simulink model "rtlsdr_datafm_image_audio"  (R2014b)
settings: Solver=ode45  StartTime=0.0  StopTime=170  RelTol=1e-3
PreLoadFcn:
  | %%%%%%%%%%%%%%%%%%%%%%%%%%%%%%%%%%%%%%%%%%%%%%%%%%%%%%%%%%%%%%%%%%%%%%%%%%%
  | % check to see if Simulink library folder is missing from the MATLAB path %
  | %%%%%%%%%%%%%%%%%%%%%%%%%%%%%%%%%%%%%%%%%%%%%%%%%%%%%%%%%%%%%%%%%%%%%%%%%%%
  | if isempty(strfind(path, 'rtlsdr_book_library'))
  | 
  |     % create error window
  |     fig_error = figure(...
  |         'Name', 'Error: RTL-SDR Book Library',...
  |         'Toolbar','none',...
  |         'MenuBar','none',...
  |         'NumberTitle','off',...
  |         'Resize','off',...
  |         'WindowStyle','modal');
  |     fig_error.Position(3) = 600;
  |     fig_error.Position(4) = 150;
  |     fig_axes = axes(...
  |         'Parent',fig_error,...
  |         'Position',[0,0,1,1],...
  |         'visible','off');
  |     % error message
  |     t_title = text(.05,.8,...
  |         'MISSING DIRECTORIES',...
  |         'FontSize',11.5);
  |     t_body = text(.075,.6,...
  |         [{'Simulink cannot find the  \it{<root>}\rm / \it{rtlsdr\_book\_library}\rm  folder in the \it{MATLAB Path}\rm.'},...
  |         {'Please set the MATLAB path following the instructions given in Exercise 2.4.'}],...
  |         'FontSize',10.5);
  |     % buttons
  |     btn_path = uicontrol(...
  |         'Parent',fig_error,...
  |         'String','Set Path Now',...
  |         'FontSize',10,...
  |         'Callback', 'pathtool; close(fig_error);',...
  |         'Position', [fig_error.Position(3)/2-210, 30, 200, 30]);
  |     btn_abort = uicontrol(...
  |         'Parent',fig_error,...
  |         'String','No thanks',...
  |         'FontSize',10,...
  |         'Callback', 'close(fig_error); abort=1;',...
  |         'Position', [fig_error.Position(3)/2+10, 30, 200, 30]);
  | 
  |     % pause to allow user to interact with error box
  |     uiwait(fig_error);
  | 
  |     % abort simulation
  |     try
  |         if abort==1
  |             set_param(gcs, 'SimulationCommand', 'stop');
  |         end
  |     end
  | 
  |     % if user has set path, allow diagram to be updated
  |     if ~exist('abort','var')
  |         % create error window
  |         fig_update = figure(...
  |             'Name', 'Update Diagram',...
  |             'Toolbar','none',...
  |             'MenuBar','none',...
  |             'NumberTitle','off',...
  |             'Resize','off');
  |         fig_update.Position(3) = 400;
  |         fig_update.Position(4) = 120;
  |         fig_axes = axes(...
  |             'Parent',fig_update,...
  |             'Position',[0,0,1,1],...
  |             'visible','off');
  |         % instruction message
  |         t_body = text(.075,.7,...
  |             'Once you have set the path, update the block diagram',...
  |             'FontSize',10.5);
  |         % button
  |         btn_update = uicontrol(...
  |             'Parent',fig_update,...
  |             'String','Update Block Diagram',...
  |             'FontSize',10,...
  |             'Callback', 'set_param(gcs,''SimulationCommand'',''update''); close(gcf)',...
  |             'Position', [fig_update.Position(3)/2-100, 30, 200, 30]);
  |     end
  | 
  |     % clear error components
  |     clear('fig_error','fig_update','fig_axes','t_title','t_body','btn_path','btn_abort','btn_update','abort');
  | 
  | end
  | %%%%%%%%%%%%%%%%%%%%%%%%%%%%%%%%%%%%%%%%%%%%%%%%%%%%%%%%%%%%%%%%%%%%%%%%%%%
undefined symbols (not defined in the file): dfilt, fdesignblkfcn, frm, gcbh, startfcn_spectrum_analyzer
libraries: simulink x5, dsparch4 x3, rtlsdr_book_library x3, dspmlti4 x2, commutil2 x2, commrfcorlib x1, dspstat3 x1, sdrrlib x1, dspsnks4 x1
CloseFcn:
  | closefcn_model;
Description:
  | Software, Simulation Examples and Design Exercises Licence Agreement
  | 
  | This license agreement refers to the simulation examples, design exercises and files,
  | and associated software MATLAB and Simulink resources that accompany the book:
  | 
  |      Title: Software Defined Radio using MATLAB & Simulink and the RTL-SDR
  |      Published by Strathclyde Academic Media, 2015
  |      Authored by Robert W. Stewart, Kenneth W. Barlee, Dale S.W. Atkinson,
  |      and Louise H. Crockett
  | 
  | and made available as a download from, www.desktopSDR.com or variously acquired
  | by other means such as via USB storage, cloud storage, disk or any other electronic
  | or optical or magnetic storage mechanism. These files and associated software may
  | be used subject to the terms of agreement of the conditions below:
  | 
  |     Copyright © 2015 Robert W. Stewart, Kenneth W. Barlee, Dale S.W. Atkinson,
  |     and Louise H. Crockett
  |     All rights reserved.
  | 
  | Redistribution and use in source and binary forms, with or without modification, are
  | permitted provided that the following conditions are met:
  | 
  |    1.  Redistributions of source code must retain the above copyright notice, this list of
  |         conditions and the following disclaimer.
  | 
  |    2.  Redistributions in binary form must reproduce the above copyright notice, this
  |         list of conditions and the following disclaimer in the documentation and/or other
  |         materials provided with the distribution.
  | 
  |    3.  Neither the name of the copyright holder nor the names of its contributors may
  |         be used to endorse or promote products derived from this software without
  |         specific prior written permission.
  | 
  |    4.  In all cases, the software is, and all modifications and derivatives of the
  |         software shall be, licensed to you solely for use in conjunction with The
  |         MathWorks, Inc. products and service offerings.
  | 
  | THIS SOFTWARE IS PROVIDED BY THE COPYRIGHT HOLDERS AND CONTRIBUTORS
  | "AS IS" AND ANY EXPRESS OR IMPLIED WARRANTIES, INCLUDING, BUT NOT LIMITED
  | TO, THE IMPLIED WARRANTIES OF MERCHANTABILITY AND FITNESS FOR A
  | PARTICULAR PURPOSE ARE DISCLAIMED. IN NO EVENT SHALL THE COPYRIGHT
  | HOLDER OR CONTRIBUTORS BE LIABLE FOR ANY DIRECT, INDIRECT, INCIDENTAL,
  | SPECIAL, EXEMPLARY, OR CONSEQUENTIAL DAMAGES (INCLUDING, BUT NOT
  | LIMITED TO, PROCUREMENT OF SUBSTITUTE GOODS OR SERVICES; LOSS OF USE,
  | DATA, OR PROFITS; OR BUSINESS INTERRUPTION) HOWEVER CAUSED AND ON ANY
  | THEORY OF LIABILITY, WHETHER IN CONTRACT, STRICT LIABILITY, OR TORT
  | (INCLUDING NEGLIGENCE OR OTHERWISE) ARISING IN ANY WAY OUT OF THE USE
  | OF THIS SOFTWARE, EVEN IF ADVISED OF THE POSSIBILITY OF SUCH DAMAGE.
  | 
  | 
  | Audio Tracks used in Simulations Examples and Design Exercises
  | 
  | The music and vocal files used within the Examples files and software within the book
  | were variously written, arranged, performed, recorded and produced by Garrey Rice,
  | Adam Struth, Jamie Struth, Iain Thistlethwaite and also Marshall Craigmyle who
  | collectively, and individually where appropriate, assert and retain all of their copyright,
  | performance and artistic rights. Permission to use and reproduce this music is
  | granted for all purposes associated with MATLAB and Simulink software and the
  | simulation examples and design exercises files that accompany this book. Requests to
  | use the music for any other purpose should be directed to: info@desktopSDR.com.
  | For information on music track names, full credits, and links to the musicians please
  | refer to www.desktopSDR.com/more/audio.
settings Model: SimulationMode=accelerator  Creator=desktopSDR Team  LastModifiedBy=desktopSDR Team
settings DataIOCC: LimitDataPoints=off  SaveOutput=off  SignalLogging=off  SaveTime=off

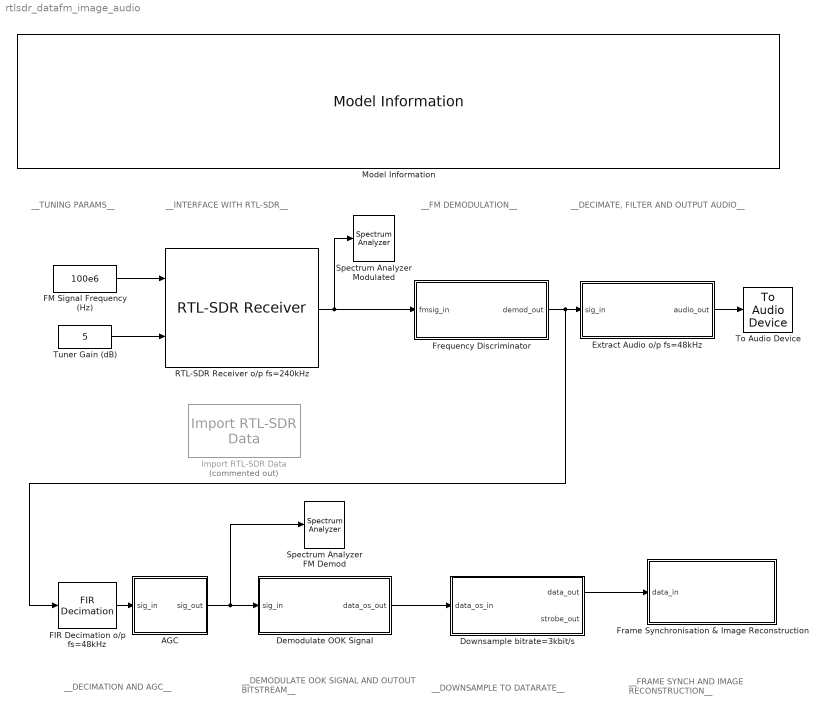
== system rtlsdr_datafm_image_audio ==
  note: __FRAME SYNCH AND
      | IMAGE RECONSTRUCTION__
  note: __FM DEMODULATION__
  note: __INTERFACE WITH RTL-SDR__
  note: __TUNING PARAMS__
  note: __DECIMATE, FILTER AND OUTPUT AUDIO__
  note: __DECIMATION AND AGC__
  note: __DOWNSAMPLE TO DATARATE__
  note: __DEMODULATE OOK SIGNAL
      | AND OUTOUT BITSTREAM__
  AGC : Subsystem
  Demodulate OOK Signal : Subsystem
  Downsample bitrate=3kbit/s : Subsystem  mask{fs=3e3}
      mask prompts: fs "Data bitrate (bit/s):"
      mask help: This block is used to downsample the received (oversampled) data back to its original bitrate. It comprises of an edge detector and a sampler.
  Extract Audio o/p fs=48kHz : Subsystem
  FIR Decimation o/p fs=48kHz : dspmlti4/FIR Decimation  h=firpm(150, [0 15e3 20e3 (240e3/2)]/(240e3/2), [1 1 0 0], [1 1],20)  D=5  filtStruct=Direct form  framing=Allow multirate processing  inputOffset=0  outputBufInitCond=0  InputProcessing=Columns as channels (frame based)  firstCoeffDataTypeStr=Inherit: Same word length as input  firstCoeffLastDataTypeStr=Inherit: Same word length as input  firstCoeffMin=[]  firstCoeffMax=[]  outputDataTypeStr=Inherit: Same as accumulator  outputLastDataTypeStr=Inherit: Same as accumulator  outputMin=[]  outputMax=[]  roundingMode=Floor  overflowMode=off  FilterSource=Specify via dialog  FilterObject=Hm_firdecim
      settings: allowOverrides=off
  "FM Signal Frequency (Hz) " : Constant  Value=100e6
  Frame Synchronisation & Image Reconstruction : Subsystem  mask(Receiver Parameter Settings){binary_len=8}
      mask prompts: binary_len "Image Pixel Bit Depth"
      mask help: The subsystem implements frame synchronisation to re-frame the received data back to its original frame structure. The preamble is then removed before the remaining header and payload data are used to recover and reconstruct the transmitted image.
      mask init:
      | try 
      |     image_receive;
      | catch ME
      |     if(strcmp(ME.identifier,'MATLAB.UndefinedFunction'))
      |         error('Unable to find "image_receive.m".');
      |     end
      |     rethrow(ME);
      | end
      mask Callback binary_len:
      | try
      |     image_receive;
      | end
  Frequency Discriminator : Subsystem
  Import RTL-SDR Data : rtlsdr_book_library/Additional Tools/Import RTL-SDR Data  Commented=on  filename=rec_data\datafm_image_audio.mat  frm_size=4096  data_type=single
  Model Information : rtlsdr_book_library/Additional Tools/Model Information/Model Information
  RTL-SDR Receiver o/p fs=240kHz : sdrrlib/RTL-SDR Receiver  SourceLibraryInfo="This block requires <a href=\"http://www.mathworks.com/hardware-support/rtl-sdr.html\">Communications System Toolbox Support Package for RTL-SDR Radio</a>"  sobjType=sdrr.internal.SDRRTLReceiverSL  IPAddress=0  dataUDPPort=-1  ctrlUDPPort=-1  subDeviceList=nosubdev  sdrBlockType=SDRBlockTypeSLT.SDRRxBlock  requester=UNUSED_BY_SFCN  sdrExecutionMode=SDRExecutionModeSLT.ExecModeHW  LostSamplesOutputPort=off  OutputDataType=single  FrameLength=4096  EnableBurstMode=off  NumFramesInBurst=20  BypassUserLogic=off  DecimatorSelect=DDC decimator  SourceSelect=RF data  SineAmplitude=16000  EnableInternalClock=off  BypassIQBalance=off  CenterFrequency=433.9e6  IFBandwidth=40e6  ADCRateSource=Dialog  ADCRate=240e3  CenterFrequencySource=Input port  GainSource=Input port  IntermediateFrequency=0  Gain=15  DecimationFactorSource=Dialog  DecimationFactor=512  RFFrequencyIsTunable=logical(1)  SampleTime=(4096)/(240e3)  IFBandwidthSource=Dialog  SineFrequency=30000  BypassDCBlockingFilter=off  IntermediateFrequencySource=Dialog  IQBalanceCoefficients=64  SkipAllHardwareResetAndInitialization=off  EnableIQCalibrationTable=on  CacheIQCalibrationTable=off  EnableOffsetTuning=off  EnableRTLAGC=off  EnableTestMode=off  EnableTunerAGC=off  FrequencyCorrectionSource=Dialog  FrequencyCorrection=0  NumMLBuffers=128  NumUSBBuffers=16  LatencyOutputPort=off  RTLCrystalFrequency=28800000  TunerCrystalFrequency=28800000
  Spectrum Analyzer Modulated : SpectrumAnalyzer  StartFcn=startfcn_spectrum_analyzer;
  Spectrum Analyzer FM Demod : SpectrumAnalyzer  StartFcn=startfcn_spectrum_analyzer;
  To Audio Device : dspsnks4/To Audio Device  deviceName=Default  inheritSampleRate=on  sampleRate=44100  deviceDatatype=Determine from input data type  autoBufferSize=on  bufferSize=4096  queueDuration=1.0  defaultOutputChannelMapping=on  outputChannelMapping=1:2  outputNumUnderrunSamples=off
  Tuner Gain (dB) : Constant  Value=5
  wires:
  Tuner Gain (dB)/1 -> RTL-SDR Receiver o/p fs=240kHz/2
  "FM Signal Frequency (Hz) "/1 -> RTL-SDR Receiver o/p fs=240kHz/1
  Extract Audio o/p fs=48kHz/1(audio_out) -> To Audio Device/1
  Downsample bitrate=3kbit/s/1(data_out) -> Frame Synchronisation & Image Reconstruction/1(data_in)
  FIR Decimation o/p fs=48kHz/1 -> AGC/1(sig_in)
  Frequency Discriminator/1(demod_out) -> FIR Decimation o/p fs=48kHz/1, Extract Audio o/p fs=48kHz/1(sig_in)
  Demodulate OOK Signal/1(data_os_out) -> Downsample bitrate=3kbit/s/1(data_os_in)
  AGC/1(sig_out) -> Demodulate OOK Signal/1(sig_in), Spectrum Analyzer FM Demod/1
  RTL-SDR Receiver o/p fs=240kHz/1 -> Spectrum Analyzer Modulated/1, Frequency Discriminator/1(fmsig_in)

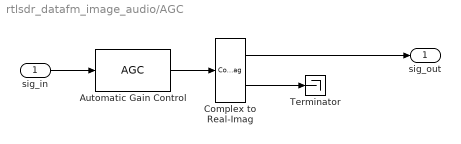
== system rtlsdr_datafm_image_audio/AGC ==
  sig_in : Inport
  Automatic Gain Control : commrfcorlib/AGC  SimulateUsing=Code generation  DetectorMethod=Rectifier  LoopMethod=Linear  UpdatePeriod=128  StepSize=0.03  MaximumGain=20  GainOutputPort=off
  Complex to Real-Imag : ComplexToRealImag
  Terminator : Terminator
  sig_out : Outport
  wires:
  Complex to Real-Imag/1 -> sig_out/1
  Automatic Gain Control/1 -> Complex to Real-Imag/1
  sig_in/1 -> Automatic Gain Control/1
  Complex to Real-Imag/2 -> Terminator/1

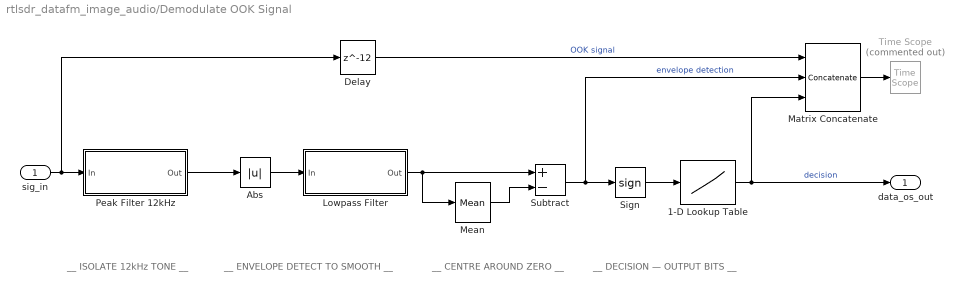
== system rtlsdr_datafm_image_audio/Demodulate OOK Signal ==
  note: __ ISOLATE 12kHz TONE __
  note: __ ENVELOPE DETECT TO SMOOTH __
  note: __ CENTRE AROUND ZERO __
  note: __ DECISION — OUTPUT BITS __
  sig_in : Inport
  1-D Lookup Table : Lookup_n-D  NumberOfTableDimensions=1  BreakpointsForDimension1=[-1,0,1]  Table=[0,0,1]  InternalRulePriority=Speed  RndMeth=Simplest  InputSameDT=on
  Abs : Abs
  Delay : Delay  DelayLength=12  InputProcessing=Columns as channels (frame based)
  Lowpass Filter : Subsystem  DialogController=fdesignblkfcn  InitFcn=fdesignblkfcn(gcbh, {'InitFcn'});  mask(Lowpass Filter){}
      mask help: Design a lowpass filter
      settings: CopyFcn=fdesignblkfcn(gcbh, {'CopyFcn'});
      mask Help: helpview(mapfilelocation('dsp'), 'dsplowpassfilter');
      mask Display: disp('Lowpass')
  Matrix Concatenate : Concatenate  NumInputs=3  Mode=Multidimensional array  ConcatenateDimension=2
  Mean : dspstat3/Mean  run=off  reset_popup=None  InputProcessing=Columns as channels (frame based)  directionMode=Each column  dimension=1  treatSBRowAsCol=on  roiEnable=off  roiType=Rectangles  roiPortion=Entire ROI  roiOutput=Individual statistics for each ROI  roiFlag=off  outputDataTypeStr=Inherit: Same as accumulator  outputLastDataTypeStr=Inherit: Same as accumulator  outputMin=[]  outputMax=[]  roundingMode=Floor  overflowMode=off
  Peak Filter 12kHz : Subsystem  DialogController=fdesignblkfcn  InitFcn=fdesignblkfcn(gcbh, {'InitFcn'});  mask(Peak/Notch Filter){}
      mask help: Design a peak/notch filter
      settings: CopyFcn=fdesignblkfcn(gcbh, {'CopyFcn'});
      mask Help: helpview(mapfilelocation('dsp'), 'dsppeaknotchfilter');
      mask Display: disp('Peak-Notch');
  Sign : Signum
  Subtract : Sum  Inputs=+-
  Time Scope : TimeScope  Commented=on  StartFcn=startfcn_time_scope  DefaultConfigurationName=spbscopes.TimeScopeBlockCfg
  data_os_out : Outport
  wires:
  Abs/1 -> Lowpass Filter/1(In)
  Lowpass Filter/1(Out) -> Subtract/1, Mean/1
  Peak Filter 12kHz/1(Out) -> Abs/1
  Sign/1 -> 1-D Lookup Table/1
  1-D Lookup Table/1 -> Matrix Concatenate/3, data_os_out/1  "decision"
  Subtract/1 -> Matrix Concatenate/2, Sign/1  "envelope detection"
  Mean/1 -> Subtract/2
  sig_in/1 -> Peak Filter 12kHz/1(In), Delay/1
  Matrix Concatenate/1 -> Time Scope/1
  Delay/1 -> Matrix Concatenate/1  "OOK signal"

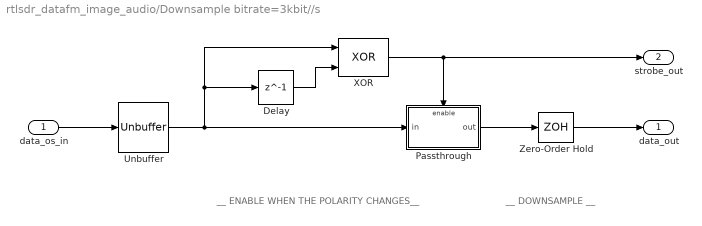
== system rtlsdr_datafm_image_audio/Downsample bitrate=3kbit//s ==
  note: __ DOWNSAMPLE __
  note: __ ENABLE WHEN THE POLARITY CHANGES__
  data_os_in : Inport
  Delay : Delay  DelayLength=1  InitialCondition=0
  Passthrough : Subsystem
  Unbuffer : Unbuffer  SampleBasedProcessing=Same as frame based
  XOR : Logic  Operator=XOR  IconShape=distinctive  AllPortsSameDT=off  OutDataTypeStr=boolean
  Zero-Order Hold : ZeroOrderHold  SampleTime=1/fs
  data_out : Outport
  strobe_out : Outport  Port=2
  wires:
  Zero-Order Hold/1 -> data_out/1
  Unbuffer/1 -> Delay/1, XOR/1, Passthrough/1(in)
  Delay/1 -> XOR/2
  XOR/1 -> strobe_out/1, Passthrough/Enable
  Passthrough/1(out) -> Zero-Order Hold/1
  data_os_in/1 -> Unbuffer/1

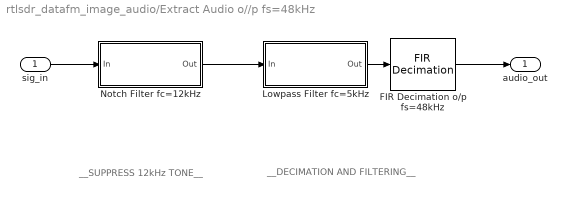
== system rtlsdr_datafm_image_audio/Extract Audio o//p fs=48kHz ==
  note: __SUPPRESS 12kHz TONE__
  note: __DECIMATION AND FILTERING__
  sig_in : Inport
  FIR Decimation o/p fs=48kHz : dspmlti4/FIR Decimation  h=firpm(150, [0 15e3 20e3 (240e3/2)]/(240e3/2), [1 1 0 0], [1 1],20)  D=5  filtStruct=Direct form  framing=Allow multirate processing  inputOffset=0  outputBufInitCond=0  InputProcessing=Columns as channels (frame based)  firstCoeffDataTypeStr=Inherit: Same word length as input  firstCoeffLastDataTypeStr=Inherit: Same word length as input  firstCoeffMin=[]  firstCoeffMax=[]  outputDataTypeStr=Inherit: Same as accumulator  outputLastDataTypeStr=Inherit: Same as accumulator  outputMin=[]  outputMax=[]  roundingMode=Floor  overflowMode=off  FilterSource=Specify via dialog  FilterObject=Hm_firdecim
      settings: allowOverrides=off
  Lowpass Filter fc=5kHz : Subsystem  DialogController=fdesignblkfcn  InitFcn=fdesignblkfcn(gcbh, {'InitFcn'});  mask(Lowpass Filter){}
      mask help: Design a lowpass filter
      settings: CopyFcn=fdesignblkfcn(gcbh, {'CopyFcn'});
      mask Help: helpview(mapfilelocation('dsp'), 'dsplowpassfilter');
      mask Display: disp('Lowpass')
  Notch Filter fc=12kHz : Subsystem  DialogController=fdesignblkfcn  InitFcn=fdesignblkfcn(gcbh, {'InitFcn'});  mask(Peak/Notch Filter){}
      mask help: Design a peak/notch filter
      settings: CopyFcn=fdesignblkfcn(gcbh, {'CopyFcn'});
      mask Help: helpview(mapfilelocation('dsp'), 'dsppeaknotchfilter');
      mask Display: disp('Peak-Notch');
  audio_out : Outport
  wires:
  sig_in/1 -> Notch Filter fc=12kHz/1(In)
  FIR Decimation o/p fs=48kHz/1 -> audio_out/1
  Lowpass Filter fc=5kHz/1(Out) -> FIR Decimation o/p fs=48kHz/1
  Notch Filter fc=12kHz/1(Out) -> Lowpass Filter fc=5kHz/1(In)

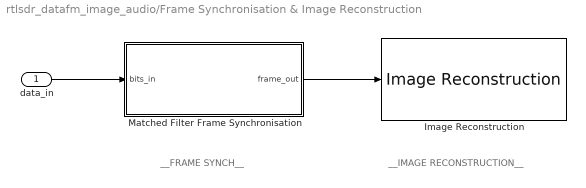
== system rtlsdr_datafm_image_audio/Frame Synchronisation & Image Reconstruction ==
  note: __FRAME SYNCH__
  note: __IMAGE RECONSTRUCTION__
  data_in : Inport
  Image Reconstruction : rtlsdr_book_library/Data Comms Sources and Sinks/Image Reconstruction
  Matched Filter Frame Synchronisation : Subsystem
  wires:
  data_in/1 -> Matched Filter Frame Synchronisation/1(bits_in)
  Matched Filter Frame Synchronisation/1(frame_out) -> Image Reconstruction/1

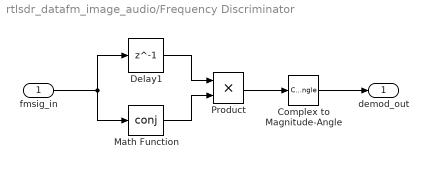
== system rtlsdr_datafm_image_audio/Frequency Discriminator ==
  fmsig_in : Inport
  Complex to Magnitude-Angle : ComplexToMagnitudeAngle  Output=Angle
  Delay1 : Delay  DelayLength=1  InitialCondition=0  InputProcessing=Columns as channels (frame based)
  Math Function : Math  Operator=conj  SaturateOnIntegerOverflow=on
  Product : Product
  demod_out : Outport
  wires:
  fmsig_in/1 -> Delay1/1, Math Function/1
  Delay1/1 -> Product/1
  Product/1 -> Complex to Magnitude-Angle/1
  Math Function/1 -> Product/2
  Complex to Magnitude-Angle/1 -> demod_out/1

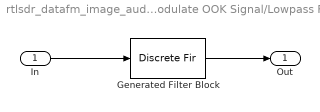
== system rtlsdr_datafm_image_audio/Demodulate OOK Signal/Lowpass Filter ==
  In : Inport
  Generated Filter Block : DiscreteFir  Tag=BlockMethodSubSystem  Coefficients=[-0.056889882382706855 0.04272587047701297 0.041865722441748722 0.046827868588471426 0.055061875523844783 0.064544738333393775 0.073956118454246697 0.082302711912541626 0.088820221635909913 0.092955621228906521 0.094371888653913771 0.092955621228906521 0.088820221635909913 0.082302711912541626 0.073956118454246697 0.064544738333393775 0.055061875523844783 0.046827868588471426 0.041865722441748722 0.04272587047701297 -0.056889882382706855]  InputProcessing=Columns as channels (frame based)
  Out : Outport
  wires:
  Generated Filter Block/1 -> Out/1
  In/1 -> Generated Filter Block/1

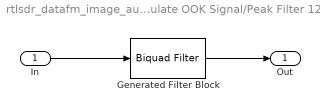
== system rtlsdr_datafm_image_audio/Demodulate OOK Signal/Peak Filter 12kHz ==
  In : Inport
  Generated Filter Block : dsparch4/Biquad Filter  Tag=BlockMethodSubSystem  IIRFiltStruct=Direct form II  CoeffSource=Specify via dialog  BiQuadCoeffs=[0.5 0 -0.5 1 0 0.66817863791929899]  a0Flag=Warning  IC=0  ICnum=0  ICden=0  InputProcessing=Columns as channels (frame based)  denAccumFracLength=30  denProdOutputFracLength=30  secondMemoryFracLength=15  roundingMode=Floor  overflowMode=off  ScaleValues=[0.33182136208070101;1]  optimizeScaleValues=off  ScaleValueMode=Specify via input port (g)  scaleValueFracLength=14  FilterSource=Specify via dialog  dfiltObjectName=dfilt.df2tsos([1 0.3 0.4],[1 0.1 0.2])
  Out : Outport
  wires:
  In/1 -> Generated Filter Block/1
  Generated Filter Block/1 -> Out/1

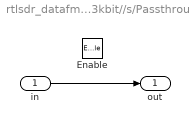
== system rtlsdr_datafm_image_audio/Downsample bitrate=3kbit//s/Passthrough ==
  in : Inport
  Enable : EnablePort
  out : Outport
  wires:
  in/1 -> out/1

== system rtlsdr_datafm_image_audio/Extract Audio o//p fs=48kHz/Lowpass Filter fc=5kHz ==
  In : Inport
  Generated Filter Block : dsparch4/Biquad Filter  Tag=BlockMethodSubSystem  IIRFiltStruct=Direct form II  CoeffSource=Specify via dialog  BiQuadCoeffs=[0.0014662393146652132 0.0029324786293304264 0.0014662393146652132 1 -1.966487213158906 0.98042551630274088;0.0022920241445179498 0.0045840482890358997 0.0022920241445179498 1 -1.9364922852784932 0.9502179867868954;0.0030462749460832615 0.006092549892166523 0.0030462749460832615 1 -1.9082335044404777 0.92175890998399401;0.0037193449217970583 0.0074386898435941165 0.0037193449217970583 1 -1.882082606511571 0.89542265659466191;0.0043036790546654565 0.0086073581093309131 0.0043036790546654565 1 -1.8583493452763198 0.87152117591334699;0.0047934341700202826 0.0095868683400405653 0.0047934341700202826 1 -1.8372871407642493 0.85030968419035424;0.0051785274900342463 0.010357054980068493 0.0051785274900342463 1 -1.819099402132154 0.83199303233021527;0.0054523704074212146 0.010904740814842429 0.0054523704074212146 1 -1.8039459107783395 0.81673213424893054;0.005590224938626656 0.011180449877253312 0.005590224938626656 1 -1.7919488018634986 0.80464999079138577;0.0054805240423490848 0.01096104808469817 0.0054805240423490848 1 -1.783197814344097 0.79583697697654865;0.0037737208845104188 0.0075474417690208377 0.0037737208845104188 1 -1.7777545856157935 0.79035516708097953;0.0031475426526353378 0.0062950853052706757 0.0031475426526353378 1 -1.7756558469630193 0.78824155273749852;0.0031542303018931022 0.0063084606037862043 0.0031542303018931022 1 -1.7762857689079308 0.78887593951847212;0.0031668170202996393 0.0063336340405992786 0.0031668170202996393 1 -1.7800598801798011 0.7926768013873734;0.0031852162333163569 0.0063704324666327139 0.0031852162333163569 1 -1.7871630750369847 0.79983034311818335;0.0032092946571374292 0.0064185893142748585 0.0032092946571374292 1 -1.7975464959615994 0.81028736089486497;0.0032388656379085386 0.0064777312758170771 0.0032388656379085386 1 -1.8111349255052718 0.82397210413382149;0.0032736806555420657 0.0065473613110841314 0.0032736806555420657 1 -1.8278230273400591 0.84077848989169335;0.0033134193124529925 0.0066268386249059849 0.0033134193124529925 1 -1.8474705515172725 0.86056527413944062;0.0033576782919589876 0.0067153565839179752 0.0033576782919589876 1 -1.8698966847064717 0.88315036195628382;0.0034059599823703102 0.0068119199647406203 0.0034059599823703102 1 -1.8948738189724748 0.90830453214031059;0.0034576617167602634 0.0069153234335205269 0.0034576617167602634 1 -1.9221211318896212 0.93574497181910243;0.0016067126669943627 0.0032134253339887254 0.0016067126669943627 1 -1.9512985141080388 0.96512916097507984;0.00080552544491969372 0.0016110508898393874 0.00080552544491969372 1 -1.9820015389165753 0.99604980635310192;0.0016828305703076845 0.003365661140615369 0.0016828305703076845 1 -1.9588485075461843 0.97273266815924442;0.0025064364169543859 0.0050128728339087717 0.0025064364169543859 1 -1.9292491998705552 0.94292356297236302;0.0032651962074720033 0.0065303924149440066 0.0032651962074720033 1 -1.9014850466339253 0.91496261965148828;0.0039502465940013855 0.0079004931880027711 0.0039502465940013855 1 -1.87591182318419 0.88920813525155573;0.0045523843762476958 0.0091047687524953916 0.0045523843762476958 1 -1.8528246319757433 0.8659573038894125;0.005055714640913209 0.010111429281826418 0.005055714640913209 1 -1.8324637859255974 0.84545214180069195;0.0054808525254435277 0.010961705050887055 0.0054808525254435277 1 -1.8150211977296618 0.82788592194304933;0.0058118949086395115 0.011623789817279023 0.0058118949086395115 1 -1.800646700304964 0.81340953923717341;0.0060459949514982715 0.012091989902996543 0.0060459949514982715 1 -1.789453871767567 0.80213737683167541;0.0051564308167370808 0.010312861633474162 0.0051564308167370808 1 -1.781525064055334 0.79415237036832775;0.0031468761340607944 0.0062937522681215888 0.0031468761340607944 1 -1.7769154336553292 0.78951006727893736;0.0031520029214611171 0.0063040058429222343 0.0031520029214611171 1 -1.7758658494881789 0.78845304374365988;0.0031631212822456067 0.0063262425644912135 0.0031631212822456067 1 -1.7788028792111099 0.79141089089695449;0.0031800779436629845 ...(+1051 chars)Flag=Warning  IC=0  ICnum=0  ICden=0  InputProcessing=Columns as channels (frame based)  denAccumFracLength=30  denProdOutputFracLength=30  secondMemoryFracLength=15  roundingMode=Floor  overflowMode=off  ScaleValues=[0.0023105936150123589;1;1;1;1;1;1;1;1;1;1;1;1;1;1;1;1;1;1;1;1;1;1;1;1;1;1;1;1;1;1;1;1;1;1;1;1;1;1;1;1;1;1;1;1;1;1;1]  optimizeScaleValues=off  ScaleValueMode=Specify via input port (g)  scaleValueFracLength=14  FilterSource=Specify via dialog  dfiltObjectName=dfilt.df2tsos([1 0.3 0.4],[1 0.1 0.2])
  Out : Outport
  wires:
  Generated Filter Block/1 -> Out/1
  In/1 -> Generated Filter Block/1

== system rtlsdr_datafm_image_audio/Extract Audio o//p fs=48kHz/Notch Filter fc=12kHz ==
  In : Inport
  Generated Filter Block : dsparch4/Biquad Filter  Tag=BlockMethodSubSystem  IIRFiltStruct=Direct form II  CoeffSource=Specify via dialog  BiQuadCoeffs=[1.051462288938775 -2 1.05146208976721 1 -1.8906743662652825 0.98217615847856421;1.0514623541957084 -2 1.0514621640514155 1 -1.878343671696399 0.98114068021814849]  a0Flag=Warning  IC=0  ICnum=0  ICden=0  InputProcessing=Columns as channels (frame based)  denAccumFracLength=30  denProdOutputFracLength=30  secondMemoryFracLength=15  roundingMode=Floor  overflowMode=off  ScaleValues=[0.0053510810621176137;1;165.93249752671582]  optimizeScaleValues=off  ScaleValueMode=Specify via input port (g)  scaleValueFracLength=14  FilterSource=Specify via dialog  dfiltObjectName=dfilt.df2tsos([1 0.3 0.4],[1 0.1 0.2])
  Out : Outport
  wires:
  Generated Filter Block/1 -> Out/1
  In/1 -> Generated Filter Block/1

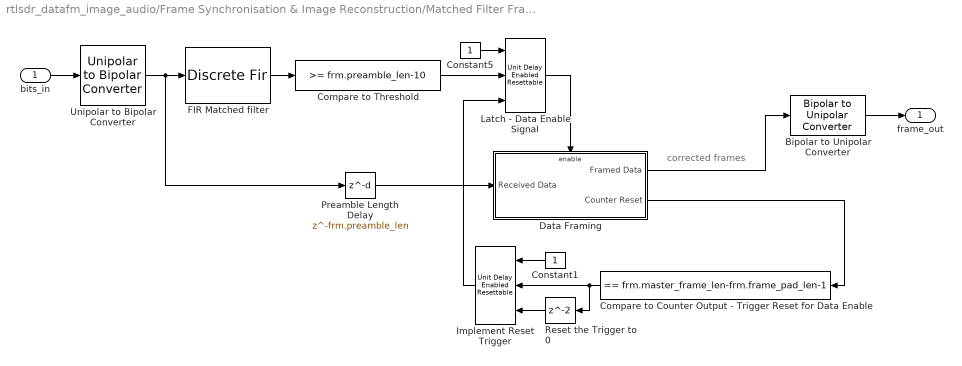
== system rtlsdr_datafm_image_audio/Frame Synchronisation & Image Reconstruction/Matched Filter Frame Synchronisation ==
  note: corrected frames
  bits_in : Inport
  Bipolar to Unipolar Converter : commutil2/Bipolar to Unipolar Converter  M=2  polarity=Positive  dataType=Inherit via internal rule
  Compare to Counter Output - Trigger Reset for Data Enable : simulink/Logic and Bit Operations/Compare To Constant  relop===  const=frm.master_frame_len-frm.frame_pad_len-1  OutDataTypeStr=boolean
  Compare to Threshold : simulink/Logic and Bit Operations/Compare To Constant  relop=>=  const=frm.preamble_len-10  OutDataTypeStr=boolean
  Constant1 : Constant
  Constant5 : Constant
  Data Framing : Subsystem
  FIR Matched filter : DiscreteFir  Coefficients=frm.filter_coeff  InputProcessing=Columns as channels (frame based)
  Implement Reset Trigger : simulink/Additional Math & Discrete/Additional Discrete/Unit Delay Enabled Resettable  vinit=0  tsamp=-1
  Latch - Data Enable Signal : simulink/Additional Math & Discrete/Additional Discrete/Unit Delay Enabled Resettable  vinit=0  tsamp=-1
  Preamble Length Delay : Delay  DelayLength=frm.preamble_len  DelayLengthUpperLimit=10000  InitialCondition=1
  Reset the Trigger to 0 : Delay  DelayLengthUpperLimit=10000  InitialCondition=0
  Unipolar to Bipolar Converter : commutil2/Unipolar to Bipolar Converter  M=2  polarity=Positive  dataType=Inherit via internal rule
  frame_out : Outport
  wires:
  Unipolar to Bipolar Converter/1 -> FIR Matched filter/1, Preamble Length Delay/1
  Bipolar to Unipolar Converter/1 -> frame_out/1
  Data Framing/2(Counter Reset) -> Compare to Counter Output - Trigger Reset for Data Enable/1
  Reset the Trigger to 0/1 -> Implement Reset Trigger/3
  FIR Matched filter/1 -> Compare to Threshold/1
  Preamble Length Delay/1 -> Data Framing/1(Received Data)
  Data Framing/1(Framed Data) -> Bipolar to Unipolar Converter/1
  Compare to Counter Output - Trigger Reset for Data Enable/1 -> Implement Reset Trigger/2, Reset the Trigger to 0/1
  Compare to Threshold/1 -> Latch - Data Enable Signal/2
  Constant1/1 -> Implement Reset Trigger/1
  bits_in/1 -> Unipolar to Bipolar Converter/1
  Constant5/1 -> Latch - Data Enable Signal/1
  Latch - Data Enable Signal/1 -> Data Framing/Enable
  Implement Reset Trigger/1 -> Latch - Data Enable Signal/3

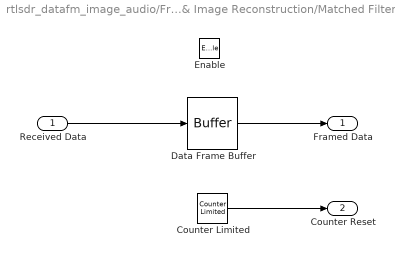
== system rtlsdr_datafm_image_audio/Frame Synchronisation & Image Reconstruction/Matched Filter Frame Synchronisation/Data Framing ==
  Received Data : Inport
  Enable : EnablePort
  Counter Limited : simulink/Sources/Counter Limited  uplimit=frm.master_frame_len-frm.frame_pad_len-1  tsamp=-1
  Data Frame Buffer : Buffer  N=frm.master_frame_len-frm.frame_pad_len  TreatMby1Signals=One channel
  Framed Data : Outport
  Counter Reset : Outport  Port=2
  wires:
  Received Data/1 -> Data Frame Buffer/1
  Data Frame Buffer/1 -> Framed Data/1
  Counter Limited/1 -> Counter Reset/1
